simulink model "PART1_protype"  (R2020a)
settings: Solver=FixedStepAuto  StartTime=0.0  StopTime=10.0  FixedStep=1e-3  RelTol=1e-3  EnableMultiTasking=on
undefined symbols (not defined in the file): D10, D11, D2, D4, D5, D7, D8, PTA0, PTA2, PTB23, PTB9, PTC3, PTD0, PTD2
libraries: frdmk64flib x7
settings Model: ExtModeTrigDuration=5  Creator=jeffl  LastModifiedBy=jeffl
settings OptimizationCC: EnhancedBackFolding=on  PassReuseOutputArgsAs=Individual arguments  ZeroExternalMemoryAtStartup=off  ZeroInternalMemoryAtStartup=off  MaxStackSize=64  OptimizeBlockOrder=speed  DifferentSizesBufferReuse=on  OptimizationCustomize=off  EfficientTunableParamExpr=on
settings DebuggingCC: ParameterTunabilityLossMsg=error
settings HardwareCC: ProdBitPerPointer=32  ProdBitPerSizeT=32  ProdBitPerPtrDiffT=32  ProdLargestAtomicInteger=Long  ProdLargestAtomicFloat=Double  ProdWordSize=32  ProdHWDeviceType=ARM Compatible->ARM Cortex
settings SFSimCC: MATLABDynamicMemAlloc=off
settings RTWCC: SystemTargetFile=ert.tlc  HardwareBoard=NXP FRDM-K64F  TemplateMakefile=ert_default_tmf  Toolchain=GNU Tools for ARM Embedded Processors
settings CodeAppCC: ForceParamTrailComments=on  IgnoreCustomStorageClasses=off  OperatorAnnotations=on  SimulinkDataObjDesc=on  SFDataObjDesc=on  InsertBlockDesc=on

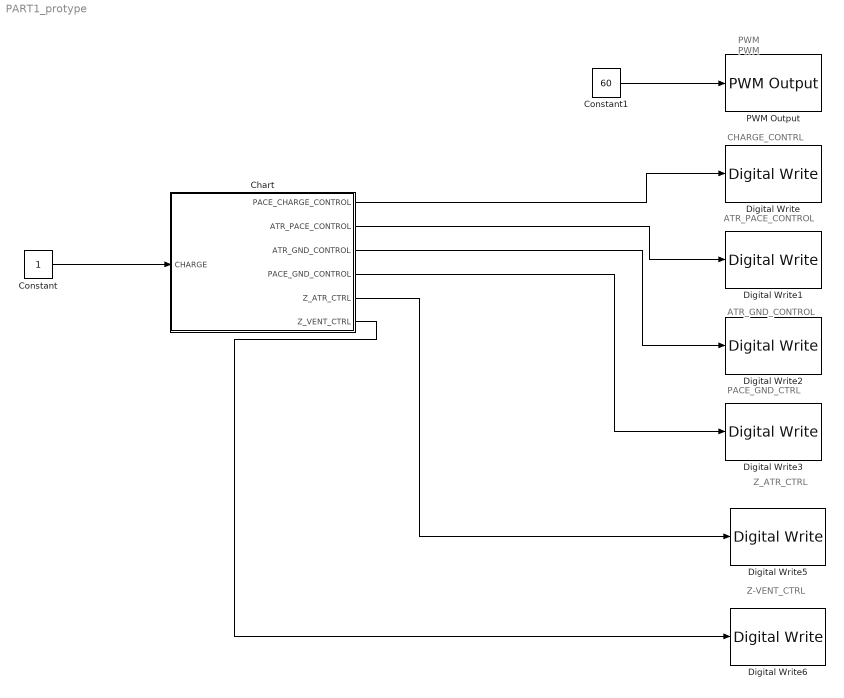
== system PART1_protype ==
  note: PACE_GND_CTRL
  note: ATR_GND_CONTROL
  note: ATR_PACE_CONTROL
  note: CHARGE_CONTRL
  note: PWM
  note: Z_ATR_CTRL
  note: Z-VENT_CTRL
  note: PWM
  Chart : Stateflow chart  TreatAsAtomicUnit=on
  Constant : Constant  OutDataTypeStr=boolean
  Constant1 : Constant  Value=60  OutDataTypeStr=double
  Digital Write : frdmk64flib/Digital Write  Whichpin=PTB9 (D2)
  Digital Write1 : frdmk64flib/Digital Write  Whichpin=PTA0 (D8)
  Digital Write2 : frdmk64flib/Digital Write  Whichpin=PTD2 (D11)
  Digital Write3 : frdmk64flib/Digital Write  Whichpin=PTD0 (D10)
  Digital Write5 : frdmk64flib/Digital Write  Whichpin=PTB23 (D4)
  Digital Write6 : frdmk64flib/Digital Write  Whichpin=PTC3 (D7)
  PWM Output : frdmk64flib/PWM Output  Whichpin=PTA2 (D5)  InitialFrequency=2000  InitialDutyCycle=0
  wires:
  Constant1/1 -> PWM Output/1
  Chart/1(PACE_CHARGE_CONTROL) -> Digital Write/1
  Chart/2(ATR_PACE_CONTROL) -> Digital Write1/1
  Chart/3(ATR_GND_CONTROL) -> Digital Write2/1
  Constant/1 -> Chart/1(CHARGE)
  Chart/4(PACE_GND_CONTROL) -> Digital Write3/1
  Chart/6(Z_VENT_CTRL) -> Digital Write6/1
  Chart/5(Z_ATR_CTRL) -> Digital Write5/1

== stateflow chart PART1_protype/Chart ==
  state CHARGE
  state Initiallizing
    entry:
    ATR_GND_CONTROL= false;
    PACE_CHARGE_CONTROL= false;
    Z_ATR_CTRL = false;
    Z_VENT_CTRL = false;
  state PACE_CONTROL
    entry:
    PACE_CHARGE_CONTROL= true;
  state ATR_PACE
    entry:
    ATR_PACE_CONTROL = true;
    PACE_GND_CONTROL= true;
  note: capaitor charged
  note: PACE COMPLETE
  state Discharge
    entry:
    ATR_GND_CONTROL = true;
  (default) -> CHARGE
  Discharge -> CHARGE : [after(500,msec)]
  CHARGE -> Initiallizing : [CHARGE ==1]
  Initiallizing -> PACE_CONTROL
  PACE_CONTROL -> ATR_PACE : [after (500,msec)]{PACE_CHARGE_CONTROL=false;}
  ATR_PACE -> Discharge : [after(10,msec)]{ATR_PACE_CONTROL = false }
  data: PACE_CHARGE_CONTROL output boolean; ATR_PACE_CONTROL output boolean; ATR_GND_CONTROL output boolean; CHARGE input boolean; PACE_GND_CONTROL output; Z_ATR_CTRL output; Z_VENT_CTRL output
